simulink model "adaptivePIDv2"  (R2024a)
settings: Solver=ode45  StartTime=0.0  StopTime=5  FixedStep=1E-4  MaxStep=1E-4  RelTol=1E-3
values from neighbouring files (symbols this model uses):
  x = [input(1);input(2);input(3)]    [Dist_observer.m]
  y = [input(4),input(5),input(6)]'    [controller.m]
undefined symbols (not defined in the file or in its folder): initial_1, observer, z
settings Model: Creator=b_ant  LastModifiedBy=b_ant
settings SolverCC: ZeroCrossAlgorithm=Adaptive
settings DebuggingCC: IgnoredZcDiagnostic=none  UnconnectedInputMsg=warning  UnconnectedOutputMsg=warning  UnconnectedLineMsg=warning
settings ModelReferenceCC: EnableRefExpFcnMdlSchedulingChecks=on
settings RTWCC: GPUComputeCapability=3.5  DLArmComputeVersion=19.05

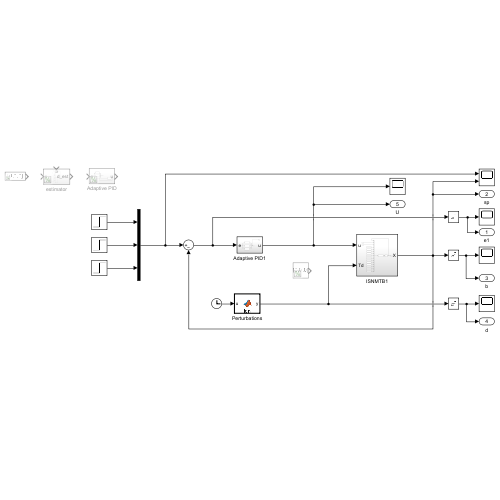
[thumbnail: Simulink's stored preview of the top-level diagram]
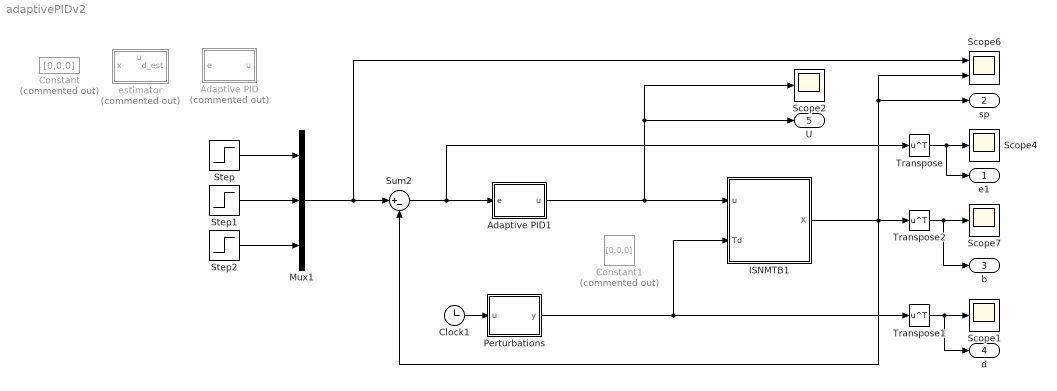
== system adaptivePIDv2 ==
  Adaptive PID : Subsystem  Commented=on
  Adaptive PID1 : Subsystem
  Clock1 : Clock
      settings: Decimation=1000
  Constant : Constant  Commented=on  Value=[0,0,0]
  Constant1 : Constant  Commented=on  Value=[0,0,0]
  ISNMTB1 : Subsystem
  Mux1 : Mux  Inputs=3
  Perturbations : MATLAB Function  TreatAsAtomicUnit=on
  Scope{1..2,4,7} (4 alike) : Scope
  Scope6 : Scope  NumInputPorts=2
  Step : Step  Time=0.1  SampleTime=0
  Step1 : Step  Time=0.1  SampleTime=0
  Step2 : Step  Time=0.1  SampleTime=0
  Sum2 : Sum  Inputs=|+-
  Transpose : Math  Operator=transpose
  Transpose1 : Math  Operator=transpose
  Transpose2 : Math  Operator=transpose
  estimator : Subsystem  Commented=on
      settings: PortSchema="{\"entries\":[{\"content\":{\"sides\":[{\"content\":{\"connectorIds\":[\"In1\"]},\"type\":\"ConnectorPlacement.EquallySpacedRectSide\",\"uuid\":\"f9e844d6-ee13-4ae8-8d73-084dc6b9c230\"},{\"content\":{\"connectorIds\":[\"Out1\"],\"side\":\"RIGHT\"},\"type\":\"ConnectorPlacement.EquallySpacedRectSide\",\"uuid\":\"c081e574-2129-4344-8b67-56cd55c23b50\"},{\"content\":{\"connectorIds\":[\"In2\"],\"side\":\"TOP\"},\"type\":\"ConnectorPlacement.EquallySpacedRectSide\",\"uuid\":\"bf6f2985-e51e-41d0-a8b1-b5505659e5f3\"},{\"content\":{\"side\":\"BOTTOM\"},\"type\":\"ConnectorPlacement.EquallySpacedRectSide\",\"uuid\":\"e1697b77-960b-449d-843b-5909cf972339\"}]},\"type\":\"ConnectorPlacement.EquallySpacedConnector\",\"uuid\":\"c9da1c41-5311-41bf-ab5b-06506202d90f\"}],\"packageUris\":[\"http://schema.mathworks.com/mf0/Connector/R2020b\"],\"version\":\"1.0\"}"
  e1 : Outport
  sp : Outport  Port=2
  b : Outport  Port=3
  d : Outport  Port=4
  U : Outport  Port=5
  wires:
  Transpose1/1 -> Scope1/1, d/1
  ISNMTB1/1(X) -> sp/1, Scope6/2, Sum2/2, Transpose2/1
  Sum2/1 -> Transpose/1, Adaptive PID1/1(e)
  Step2/1 -> Mux1/3
  Transpose2/1 -> Scope7/1, b/1
  Step1/1 -> Mux1/2
  Clock1/1 -> Perturbations/1(u)
  Transpose/1 -> e1/1, Scope4/1
  Step/1 -> Mux1/1
  Mux1/1 -> Sum2/1, Scope6/1
  Perturbations/1(y) -> ISNMTB1/2(Td), Transpose1/1
  Adaptive PID1/1(u) -> U/1, Scope2/1, ISNMTB1/1(u)

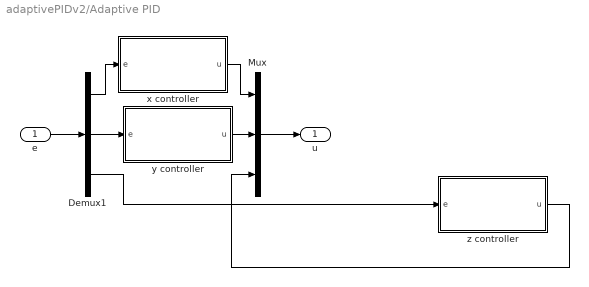
== system adaptivePIDv2/Adaptive PID ==
  e : Inport
  Demux1 : Demux  Outputs=3
  Mux : Mux  Inputs=3
  x controller : Subsystem
  y controller : Subsystem
  z controller : Subsystem
  u : Outport
  wires:
  z controller/1(u) -> Mux/3
  Demux1/2 -> y controller/1(e)
  x controller/1(u) -> Mux/1
  e/1 -> Demux1/1
  y controller/1(u) -> Mux/2
  Demux1/3 -> z controller/1(e)
  Demux1/1 -> x controller/1(e)
  Mux/1 -> u/1

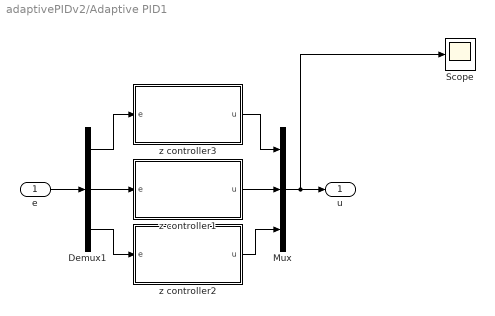
== system adaptivePIDv2/Adaptive PID1 ==
  e : Inport
  Demux1 : Demux  Outputs=3
  Mux : Mux  Inputs=3
  Scope : Scope
  z controller1 : Subsystem
  z controller2 : Subsystem
  z controller3 : Subsystem
  u : Outport
  wires:
  Demux1/2 -> z controller1/1(e)
  z controller3/1(u) -> Mux/1
  e/1 -> Demux1/1
  Demux1/1 -> z controller3/1(e)
  Mux/1 -> Scope/1, u/1
  Demux1/3 -> z controller2/1(e)
  z controller1/1(u) -> Mux/2
  z controller2/1(u) -> Mux/3

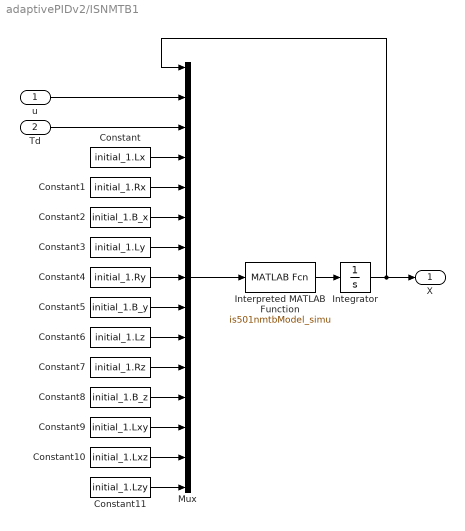
== system adaptivePIDv2/ISNMTB1 ==
  u : Inport
  Td : Inport  Port=2
  Constant : Constant  Value=initial_1.Lx
  Constant1 : Constant  Value=initial_1.Rx
  Constant10 : Constant  Value=initial_1.Lxz
  Constant11 : Constant  Value=initial_1.Lzy
  Constant2 : Constant  Value=initial_1.B_x
  Constant3 : Constant  Value=initial_1.Ly
  Constant4 : Constant  Value=initial_1.Ry
  Constant5 : Constant  Value=initial_1.B_y
  Constant6 : Constant  Value=initial_1.Lz
  Constant7 : Constant  Value=initial_1.Rz
  Constant8 : Constant  Value=initial_1.B_z
  Constant9 : Constant  Value=initial_1.Lxy
  Integrator : Integrator  InitialCondition=[3.249E4, -2.265E4, 3.655E4]
  Interpreted MATLAB Function : MATLABFcn  MATLABFcn=is501nmtbModel_simu
  Mux : Mux  Inputs=15
  X : Outport
  wires:
  Interpreted MATLAB Function/1 -> Integrator/1
  Integrator/1 -> X/1, Mux/1
  Mux/1 -> Interpreted MATLAB Function/1
  u/1 -> Mux/2
  Td/1 -> Mux/3
  Constant/1 -> Mux/4
  Constant1/1 -> Mux/5
  Constant2/1 -> Mux/6
  Constant3/1 -> Mux/7
  Constant4/1 -> Mux/8
  Constant5/1 -> Mux/9
  Constant6/1 -> Mux/10
  Constant7/1 -> Mux/11
  Constant8/1 -> Mux/12
  Constant9/1 -> Mux/13
  Constant10/1 -> Mux/14
  Constant11/1 -> Mux/15

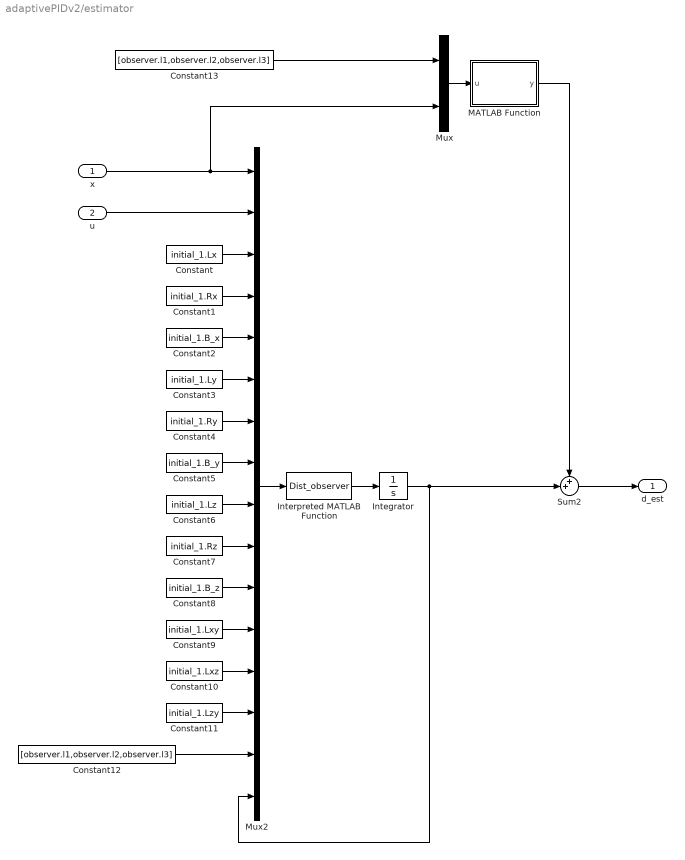
== system adaptivePIDv2/estimator ==
  x : Inport
  u : Inport  Port=2
  Constant : Constant  Value=initial_1.Lx
  Constant1 : Constant  Value=initial_1.Rx
  Constant10 : Constant  Value=initial_1.Lxz
  Constant11 : Constant  Value=initial_1.Lzy
  Constant12 : Constant  Value=[observer.l1,observer.l2,observer.l3]
  Constant13 : Constant  Value=[observer.l1,observer.l2,observer.l3]
  Constant2 : Constant  Value=initial_1.B_x
  Constant3 : Constant  Value=initial_1.Ly
  Constant4 : Constant  Value=initial_1.Ry
  Constant5 : Constant  Value=initial_1.B_y
  Constant6 : Constant  Value=initial_1.Lz
  Constant7 : Constant  Value=initial_1.Rz
  Constant8 : Constant  Value=initial_1.B_z
  Constant9 : Constant  Value=initial_1.Lxy
  Integrator : Integrator  InitialCondition=[0,0,0]
  Interpreted MATLAB Function : MATLABFcn  MATLABFcn=Dist_observer
  MATLAB Function : MATLAB Function  TreatAsAtomicUnit=on
  Mux : Mux  Inputs=2
  Mux2 : Mux  Inputs=16
  Sum2 : Sum  Inputs=++|
  d_est : Outport
  wires:
  Constant6/1 -> Mux2/9
  MATLAB Function/1(y) -> Sum2/1
  Constant10/1 -> Mux2/13
  Integrator/1 -> Sum2/2, Mux2/16
  Interpreted MATLAB Function/1 -> Integrator/1
  Constant2/1 -> Mux2/5
  Constant4/1 -> Mux2/7
  Constant7/1 -> Mux2/10
  Mux2/1 -> Interpreted MATLAB Function/1
  Constant11/1 -> Mux2/14
  Constant8/1 -> Mux2/11
  Constant1/1 -> Mux2/4
  Constant3/1 -> Mux2/6
  Constant/1 -> Mux2/3
  Constant9/1 -> Mux2/12
  Constant5/1 -> Mux2/8
  Constant12/1 -> Mux2/15
  u/1 -> Mux2/2
  Sum2/1 -> d_est/1
  Constant13/1 -> Mux/1
  Mux/1 -> MATLAB Function/1(u)
  x/1 -> Mux/2, Mux2/1

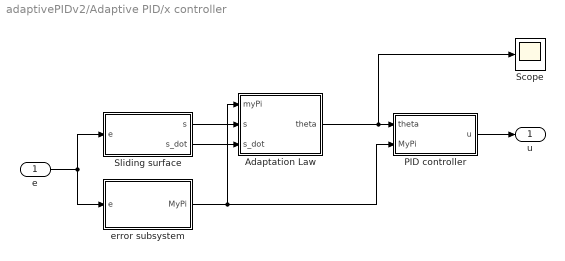
== system adaptivePIDv2/Adaptive PID/x controller ==
  e : Inport
  Adaptation Law : Subsystem  mask{alpha=x.alpha, beta=x.beta, epsilon=x.epsilon, n=x.n, kd0=x.kd_init, ki0=x.ki_init, kp0=x.kp_init}
      mask prompts: kd0 "kd_0:"; ki0 "ki_0:"; kp0 "kp_0:"
      mask TypeOptions alpha: alpha/Value
      mask TypeOptions beta: beta/Value
      mask TypeOptions epsilon: epsilon/Value
      mask TypeOptions n: n/Value
      mask TypeOptions kd0: kd0/Value
      mask TypeOptions ki0: ki0/Value
      mask TypeOptions kp0: kp0/Value
  PID controller : Subsystem
  Scope : Scope
  Sliding surface : Subsystem  mask{Gain=x.lambda}
      mask prompts: Gain "Simulink:blkprm_prompts:GainGain"
      mask TypeOptions Gain: Gain/Gain
      mask DialogControl Gain Prompt: Gain:
  error subsystem : Subsystem
  u : Outport
  wires:
  Sliding surface/1(s) -> Adaptation Law/2(s)
  Sliding surface/2(s_dot) -> Adaptation Law/3(s_dot)
  PID controller/1(u) -> u/1
  error subsystem/1(MyPi) -> PID controller/2(MyPi), Adaptation Law/1(myPi)
  e/1 -> Sliding surface/1(e), error subsystem/1(e)
  Adaptation Law/1(theta) -> Scope/1, PID controller/1(theta)

== system adaptivePIDv2/Adaptive PID/y controller ==
  e : Inport
  Adaptation Law : Subsystem  mask{alpha=y.alpha, beta=y.beta, epsilon=y.epsilon, n=y.n, kd0=y.kd_init, ki0=y.ki_init, kp0=y.kp_init}
      mask prompts: kd0 "kd_0:"; ki0 "ki_0:"; kp0 "kp_0:"
      mask TypeOptions alpha: alpha/Value
      mask TypeOptions beta: beta/Value
      mask TypeOptions epsilon: epsilon/Value
      mask TypeOptions n: n/Value
      mask TypeOptions kd0: kd0/Value
      mask TypeOptions ki0: ki0/Value
      mask TypeOptions kp0: kp0/Value
  PID controller : Subsystem
  Scope : Scope
  Sliding surface : Subsystem  mask{Gain=y.lambda}
      mask prompts: Gain "Simulink:blkprm_prompts:GainGain"
      mask TypeOptions Gain: Gain/Gain
      mask DialogControl Gain Prompt: Gain:
  error subsystem : Subsystem
  u : Outport
  wires:
  e/1 -> Sliding surface/1(e), error subsystem/1(e)
  error subsystem/1(MyPi) -> Adaptation Law/1(myPi), PID controller/2(MyPi)
  Adaptation Law/1(theta) -> PID controller/1(theta), Scope/1
  PID controller/1(u) -> u/1
  Sliding surface/2(s_dot) -> Adaptation Law/3(s_dot)
  Sliding surface/1(s) -> Adaptation Law/2(s)

== system adaptivePIDv2/Adaptive PID/z controller ==
  e : Inport
  Adaptation Law : Subsystem  mask{alpha=z.alpha, beta=z.beta, epsilon=z.epsilon, n=z.n, kd0=z.kd_init, ki0=z.ki_init, kp0=z.kp_init}
      mask prompts: kd0 "kd_0:"; ki0 "ki_0:"; kp0 "kp_0:"
      mask TypeOptions alpha: alpha/Value
      mask TypeOptions beta: beta/Value
      mask TypeOptions epsilon: epsilon/Value
      mask TypeOptions n: n/Value
      mask TypeOptions kd0: kd0/Value
      mask TypeOptions ki0: ki0/Value
      mask TypeOptions kp0: kp0/Value
  PID controller : Subsystem
  Scope : Scope
  Sliding surface : Subsystem  mask{Gain=z.lambda}
      mask prompts: Gain "Simulink:blkprm_prompts:GainGain"
      mask TypeOptions Gain: Gain/Gain
      mask DialogControl Gain Prompt: Gain:
  error subsystem : Subsystem
  u : Outport
  wires:
  Sliding surface/1(s) -> Adaptation Law/2(s)
  Sliding surface/2(s_dot) -> Adaptation Law/3(s_dot)
  PID controller/1(u) -> u/1
  Adaptation Law/1(theta) -> Scope/1, PID controller/1(theta)
  error subsystem/1(MyPi) -> PID controller/2(MyPi), Adaptation Law/1(myPi)
  e/1 -> error subsystem/1(e), Sliding surface/1(e)

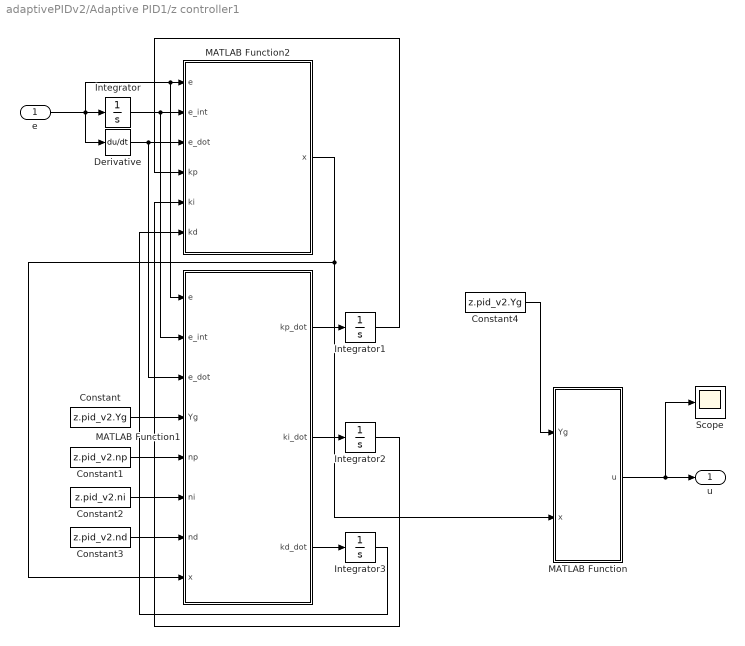
== system adaptivePIDv2/Adaptive PID1/z controller1 ==
  e : Inport
  Constant : Constant  Value=z.pid_v2.Yg
  Constant1 : Constant  Value=z.pid_v2.np
  Constant2 : Constant  Value=z.pid_v2.ni
  Constant3 : Constant  Value=z.pid_v2.nd
  Constant4 : Constant  Value=z.pid_v2.Yg
  Derivative : Derivative
  Integrator : Integrator
  Integrator1 : Integrator  InitialCondition=y.PID.Kp
  Integrator2 : Integrator  InitialCondition=y.PID.Ki
  Integrator3 : Integrator  InitialCondition=y.PID.Kd
  MATLAB Function : MATLAB Function  TreatAsAtomicUnit=on
  MATLAB Function1 : MATLAB Function  TreatAsAtomicUnit=on
  MATLAB Function2 : MATLAB Function  TreatAsAtomicUnit=on
  Scope : Scope
  u : Outport
  wires:
  e/1 -> Derivative/1, Integrator/1, MATLAB Function1/1(e), MATLAB Function2/1(e)
  Constant/1 -> MATLAB Function1/4(Yg)
  Constant1/1 -> MATLAB Function1/5(np)
  Constant2/1 -> MATLAB Function1/6(ni)
  Constant3/1 -> MATLAB Function1/7(nd)
  Constant4/1 -> MATLAB Function/1(Yg)
  MATLAB Function1/1(kp_dot) -> Integrator1/1
  MATLAB Function1/2(ki_dot) -> Integrator2/1
  MATLAB Function1/3(kd_dot) -> Integrator3/1
  Integrator/1 -> MATLAB Function1/2(e_int), MATLAB Function2/2(e_int)
  Derivative/1 -> MATLAB Function1/3(e_dot), MATLAB Function2/3(e_dot)
  MATLAB Function2/1(x) -> MATLAB Function/2(x), MATLAB Function1/8(x)
  Integrator1/1 -> MATLAB Function2/4(kp)
  Integrator2/1 -> MATLAB Function2/5(ki)
  Integrator3/1 -> MATLAB Function2/6(kd)
  MATLAB Function/1(u) -> Scope/1, u/1

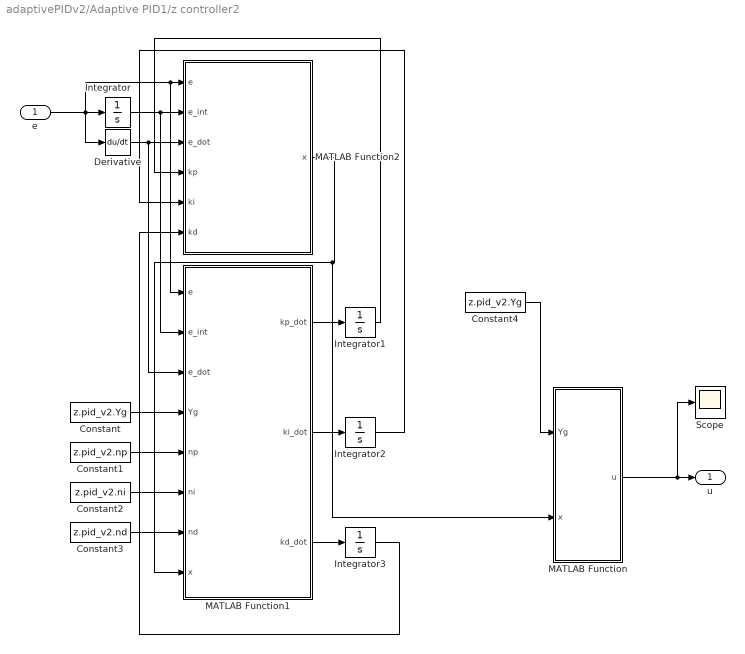
== system adaptivePIDv2/Adaptive PID1/z controller2 ==
  e : Inport
  Constant : Constant  Value=z.pid_v2.Yg
  Constant1 : Constant  Value=z.pid_v2.np
  Constant2 : Constant  Value=z.pid_v2.ni
  Constant3 : Constant  Value=z.pid_v2.nd
  Constant4 : Constant  Value=z.pid_v2.Yg
  Derivative : Derivative
  Integrator : Integrator
  Integrator1 : Integrator  InitialCondition=z.PID.Kp
  Integrator2 : Integrator  InitialCondition=z.PID.Ki
  Integrator3 : Integrator  InitialCondition=z.PID.Kd
  MATLAB Function : MATLAB Function  TreatAsAtomicUnit=on
  MATLAB Function1 : MATLAB Function  TreatAsAtomicUnit=on
  MATLAB Function2 : MATLAB Function  TreatAsAtomicUnit=on
  Scope : Scope
  u : Outport
  wires:
  e/1 -> Derivative/1, Integrator/1, MATLAB Function1/1(e), MATLAB Function2/1(e)
  Constant/1 -> MATLAB Function1/4(Yg)
  Constant1/1 -> MATLAB Function1/5(np)
  Constant2/1 -> MATLAB Function1/6(ni)
  Constant3/1 -> MATLAB Function1/7(nd)
  Constant4/1 -> MATLAB Function/1(Yg)
  MATLAB Function1/1(kp_dot) -> Integrator1/1
  MATLAB Function1/2(ki_dot) -> Integrator2/1
  MATLAB Function1/3(kd_dot) -> Integrator3/1
  Integrator/1 -> MATLAB Function1/2(e_int), MATLAB Function2/2(e_int)
  Derivative/1 -> MATLAB Function1/3(e_dot), MATLAB Function2/3(e_dot)
  MATLAB Function2/1(x) -> MATLAB Function/2(x), MATLAB Function1/8(x)
  Integrator1/1 -> MATLAB Function2/4(kp)
  Integrator2/1 -> MATLAB Function2/5(ki)
  Integrator3/1 -> MATLAB Function2/6(kd)
  MATLAB Function/1(u) -> Scope/1, u/1

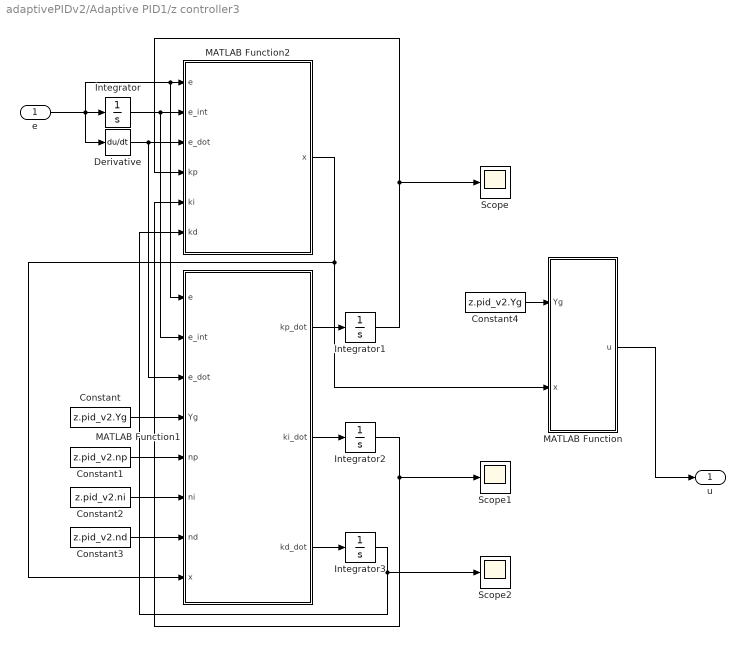
== system adaptivePIDv2/Adaptive PID1/z controller3 ==
  e : Inport
  Constant : Constant  Value=z.pid_v2.Yg
  Constant1 : Constant  Value=z.pid_v2.np
  Constant2 : Constant  Value=z.pid_v2.ni
  Constant3 : Constant  Value=z.pid_v2.nd
  Constant4 : Constant  Value=z.pid_v2.Yg
  Derivative : Derivative
  Integrator : Integrator
  Integrator1 : Integrator  InitialCondition=x.PID.Kp
  Integrator2 : Integrator  InitialCondition=x.PID.Ki
  Integrator3 : Integrator  InitialCondition=x.PID.Kd
  MATLAB Function : MATLAB Function  TreatAsAtomicUnit=on
  MATLAB Function1 : MATLAB Function  TreatAsAtomicUnit=on
  MATLAB Function2 : MATLAB Function  TreatAsAtomicUnit=on
  Scope : Scope
  Scope1 : Scope
  Scope2 : Scope
  u : Outport
  wires:
  e/1 -> Derivative/1, Integrator/1, MATLAB Function1/1(e), MATLAB Function2/1(e)
  Constant/1 -> MATLAB Function1/4(Yg)
  Constant1/1 -> MATLAB Function1/5(np)
  Constant2/1 -> MATLAB Function1/6(ni)
  Constant3/1 -> MATLAB Function1/7(nd)
  Constant4/1 -> MATLAB Function/1(Yg)
  MATLAB Function1/1(kp_dot) -> Integrator1/1
  MATLAB Function1/2(ki_dot) -> Integrator2/1
  MATLAB Function1/3(kd_dot) -> Integrator3/1
  Integrator/1 -> MATLAB Function1/2(e_int), MATLAB Function2/2(e_int)
  Derivative/1 -> MATLAB Function1/3(e_dot), MATLAB Function2/3(e_dot)
  MATLAB Function2/1(x) -> MATLAB Function/2(x), MATLAB Function1/8(x)
  Integrator1/1 -> Scope/1, MATLAB Function2/4(kp)
  Integrator2/1 -> MATLAB Function2/5(ki), Scope1/1
  Integrator3/1 -> Scope2/1, MATLAB Function2/6(kd)
  MATLAB Function/1(u) -> u/1

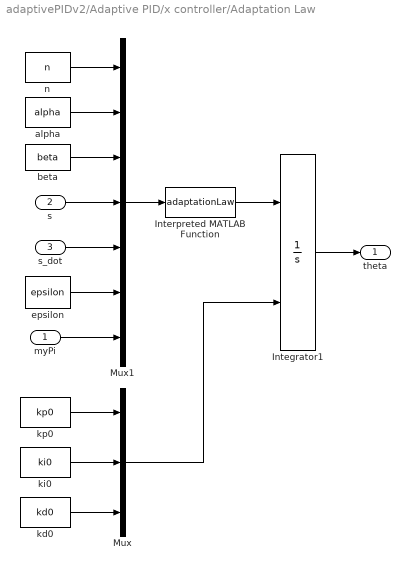
== system adaptivePIDv2/Adaptive PID/x controller/Adaptation Law ==
  myPi : Inport
  s : Inport  Port=2
  s_dot : Inport  Port=3
  Integrator1 : Integrator  InitialConditionSource=external  InitialCondition=[1.460477259865257e-04,6.548069875818259e-05,0]
  Interpreted MATLAB Function : MATLABFcn  MATLABFcn=adaptationLaw
  Mux : Mux  Inputs=3
  Mux1 : Mux  Inputs=7
  alpha : Constant  Value=alpha
  beta : Constant  Value=beta
  epsilon : Constant  Value=epsilon
  kd0 : Constant  Value=kd0
  ki0 : Constant  Value=ki0
  kp0 : Constant  Value=kp0
  n : Constant  Value=n
  theta : Outport
  wires:
  alpha/1 -> Mux1/2
  Interpreted MATLAB Function/1 -> Integrator1/1
  myPi/1 -> Mux1/7
  s/1 -> Mux1/4
  epsilon/1 -> Mux1/6
  Integrator1/1 -> theta/1
  s_dot/1 -> Mux1/5
  beta/1 -> Mux1/3
  Mux1/1 -> Interpreted MATLAB Function/1
  n/1 -> Mux1/1
  ki0/1 -> Mux/2
  Mux/1 -> Integrator1/2
  kp0/1 -> Mux/1
  kd0/1 -> Mux/3

== system adaptivePIDv2/Adaptive PID/x controller/PID controller ==
  theta : Inport
  MyPi : Inport  Port=2
  Interpreted MATLAB Function1 : MATLABFcn  MATLABFcn=controlLaw  OutputDimensions=1
  Mux2 : Mux  Inputs=2
  u : Outport
  wires:
  Mux2/1 -> Interpreted MATLAB Function1/1
  theta/1 -> Mux2/1
  Interpreted MATLAB Function1/1 -> u/1
  MyPi/1 -> Mux2/2

== system adaptivePIDv2/Adaptive PID/x controller/Sliding surface ==
  note: s
  note: e
  e : Inport
  Add : Sum
  Derivative : Derivative
  Derivative1 : Derivative
  Gain : Gain  Gain=Gain
  s : Outport
  s_dot : Outport  Port=2
  wires:
  Add/1 -> s/1, Derivative/1
  Gain/1 -> Add/1
  e/1 -> Derivative1/1, Gain/1
  Derivative1/1 -> Add/2
  Derivative/1 -> s_dot/1

== system adaptivePIDv2/Adaptive PID/x controller/error subsystem ==
  e : Inport
  Derivative : Derivative
  Integrator : Integrator
  Mux : Mux  Inputs=3
  MyPi : Outport
  wires:
  e/1 -> Derivative/1, Mux/1, Integrator/1
  Integrator/1 -> Mux/2
  Mux/1 -> MyPi/1
  Derivative/1 -> Mux/3

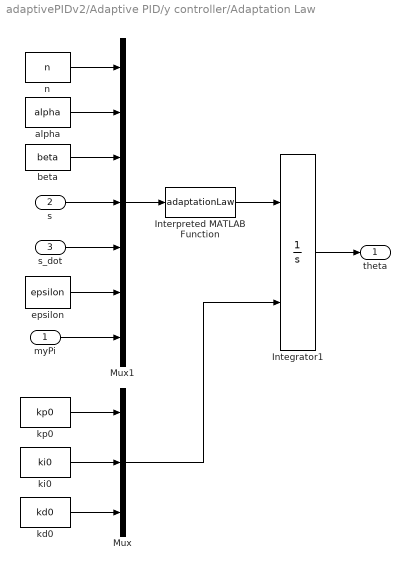
== system adaptivePIDv2/Adaptive PID/y controller/Adaptation Law ==
  myPi : Inport
  s : Inport  Port=2
  s_dot : Inport  Port=3
  Integrator1 : Integrator  InitialConditionSource=external  InitialCondition=[1.460477259865257e-04,6.548069875818259e-05,0]
  Interpreted MATLAB Function : MATLABFcn  MATLABFcn=adaptationLaw
  Mux : Mux  Inputs=3
  Mux1 : Mux  Inputs=7
  alpha : Constant  Value=alpha
  beta : Constant  Value=beta
  epsilon : Constant  Value=epsilon
  kd0 : Constant  Value=kd0
  ki0 : Constant  Value=ki0
  kp0 : Constant  Value=kp0
  n : Constant  Value=n
  theta : Outport
  wires:
  kd0/1 -> Mux/3
  kp0/1 -> Mux/1
  Mux/1 -> Integrator1/2
  ki0/1 -> Mux/2
  n/1 -> Mux1/1
  Mux1/1 -> Interpreted MATLAB Function/1
  beta/1 -> Mux1/3
  s_dot/1 -> Mux1/5
  Integrator1/1 -> theta/1
  epsilon/1 -> Mux1/6
  s/1 -> Mux1/4
  myPi/1 -> Mux1/7
  Interpreted MATLAB Function/1 -> Integrator1/1
  alpha/1 -> Mux1/2

== system adaptivePIDv2/Adaptive PID/y controller/PID controller ==
  theta : Inport
  MyPi : Inport  Port=2
  Interpreted MATLAB Function1 : MATLABFcn  MATLABFcn=controlLaw  OutputDimensions=1
  Mux2 : Mux  Inputs=2
  u : Outport
  wires:
  MyPi/1 -> Mux2/2
  Interpreted MATLAB Function1/1 -> u/1
  theta/1 -> Mux2/1
  Mux2/1 -> Interpreted MATLAB Function1/1

== system adaptivePIDv2/Adaptive PID/y controller/Sliding surface ==
  note: e
  note: s
  e : Inport
  Add : Sum
  Derivative : Derivative
  Derivative1 : Derivative
  Gain : Gain  Gain=Gain
  s : Outport
  s_dot : Outport  Port=2
  wires:
  Derivative/1 -> s_dot/1
  Derivative1/1 -> Add/2
  e/1 -> Derivative1/1, Gain/1
  Gain/1 -> Add/1
  Add/1 -> s/1, Derivative/1

== system adaptivePIDv2/Adaptive PID/y controller/error subsystem ==
  e : Inport
  Derivative : Derivative
  Integrator : Integrator
  Mux : Mux  Inputs=3
  MyPi : Outport
  wires:
  Derivative/1 -> Mux/3
  Mux/1 -> MyPi/1
  Integrator/1 -> Mux/2
  e/1 -> Derivative/1, Integrator/1, Mux/1

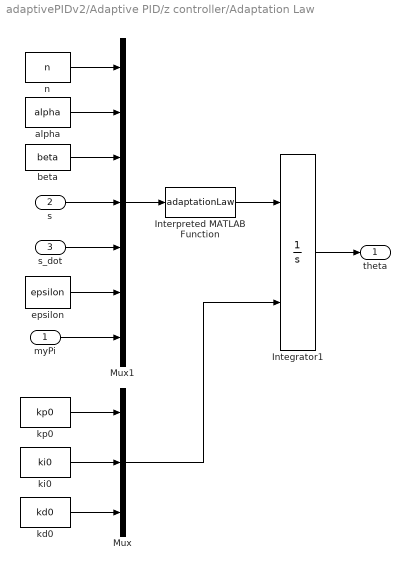
== system adaptivePIDv2/Adaptive PID/z controller/Adaptation Law ==
  myPi : Inport
  s : Inport  Port=2
  s_dot : Inport  Port=3
  Integrator1 : Integrator  InitialConditionSource=external  InitialCondition=[1.460477259865257e-04,6.548069875818259e-05,0]
  Interpreted MATLAB Function : MATLABFcn  MATLABFcn=adaptationLaw
  Mux : Mux  Inputs=3
  Mux1 : Mux  Inputs=7
  alpha : Constant  Value=alpha
  beta : Constant  Value=beta
  epsilon : Constant  Value=epsilon
  kd0 : Constant  Value=kd0
  ki0 : Constant  Value=ki0
  kp0 : Constant  Value=kp0
  n : Constant  Value=n
  theta : Outport
  wires:
  alpha/1 -> Mux1/2
  Interpreted MATLAB Function/1 -> Integrator1/1
  myPi/1 -> Mux1/7
  s/1 -> Mux1/4
  epsilon/1 -> Mux1/6
  Integrator1/1 -> theta/1
  s_dot/1 -> Mux1/5
  beta/1 -> Mux1/3
  Mux1/1 -> Interpreted MATLAB Function/1
  n/1 -> Mux1/1
  ki0/1 -> Mux/2
  Mux/1 -> Integrator1/2
  kp0/1 -> Mux/1
  kd0/1 -> Mux/3

== system adaptivePIDv2/Adaptive PID/z controller/PID controller ==
  theta : Inport
  MyPi : Inport  Port=2
  Interpreted MATLAB Function1 : MATLABFcn  MATLABFcn=controlLaw  OutputDimensions=1
  Mux2 : Mux  Inputs=2
  u : Outport
  wires:
  Mux2/1 -> Interpreted MATLAB Function1/1
  theta/1 -> Mux2/1
  Interpreted MATLAB Function1/1 -> u/1
  MyPi/1 -> Mux2/2

== system adaptivePIDv2/Adaptive PID/z controller/Sliding surface ==
  note: s
  note: e
  e : Inport
  Add : Sum
  Derivative : Derivative
  Derivative1 : Derivative
  Gain : Gain  Gain=Gain
  s : Outport
  s_dot : Outport  Port=2
  wires:
  Add/1 -> s/1, Derivative/1
  Gain/1 -> Add/1
  e/1 -> Derivative1/1, Gain/1
  Derivative1/1 -> Add/2
  Derivative/1 -> s_dot/1

== system adaptivePIDv2/Adaptive PID/z controller/error subsystem ==
  e : Inport
  Derivative : Derivative
  Integrator : Integrator
  Mux : Mux  Inputs=3
  MyPi : Outport
  wires:
  e/1 -> Derivative/1, Mux/1, Integrator/1
  Integrator/1 -> Mux/2
  Mux/1 -> MyPi/1
  Derivative/1 -> Mux/3

== matlab function adaptivePIDv2/Adaptive PID1/z controller3/MATLAB Function2 ==
  data: e input; x output; e_int input; e_dot input; kp input; ki input; kd input
function x = myPidFun(e,e_int,e_dot,kp,ki,kd)
   x = kp*e+ki*e_int+kd*e_dot;
end

== matlab function adaptivePIDv2/Adaptive PID1/z controller2/MATLAB Function1 ==
  data: e input; kp_dot output; e_int input; e_dot input; Yg input; np input; ni input; nd input; ki_dot output; kd_dot output; x input
function [kp_dot,ki_dot,kd_dot] = neuronalPID(e,e_int,e_dot,Yg,np,ni,nd,x)
%e = entr(1);
%e_int = entr(2);
%e_dot = entr(3);
%x =  entr(4);
%Yg =  entr(5);
%np =  entr(6);
%ni =  entr(7);
%nd =  entr(8);
%kp_old
%ki_old
%kd_old 

kp_dot = np*e*e*sigmoid_dot(x, Yg);
ki_dot = ni*e*e_int*sigmoid_dot(x, Yg);
kd_dot = nd*e*e_dot*sigmoid_dot(x, Yg);
end

function f_dot = sigmoid_dot(x, Yg)
    f_dot = 4*exp(-x*Yg)/(1+exp(-x*Yg))^2;
end

== matlab function adaptivePIDv2/Adaptive PID1/z controller2/MATLAB Function2 ==
  data: e input; x output; e_int input; e_dot input; kp input; ki input; kd input
function x = myPidFun(e,e_int,e_dot,kp,ki,kd)
   x = kp*e+ki*e_int+kd*e_dot;
end

== matlab function adaptivePIDv2/Perturbations ==
  data: u input; y output
function y = fcn(u)
y= [2.522*sin(2*pi*4.788E-3*u)+3.249E04;
   -5.174*sin(2*pi*7.481E-3*u)-2.265E04;
    3.359*sin(2*pi*8.378E-3*u)+3.655E04];
end

== matlab function adaptivePIDv2/Adaptive PID1/z controller1/MATLAB Function ==
  data: Yg input; u output; x input
function u = fcn(Yg, x)
    u=sigmoid(x,Yg);
end

function f = sigmoid(x,Yg)
    f = 2/Yg * (1-exp(-x*Yg))/(1+exp(-x*Yg));
end

== matlab function adaptivePIDv2/estimator/MATLAB Function ==
  data: u input; y output
function y = fcn(u)
l = diag([u(1),u(2),u(3)]);
x = [u(4);u(5);u(6)];

y = l*x;
end

== matlab function adaptivePIDv2/Adaptive PID1/z controller1/MATLAB Function1 ==
  data: e input; kp_dot output; e_int input; e_dot input; Yg input; np input; ni input; nd input; ki_dot output; kd_dot output; x input
function [kp_dot,ki_dot,kd_dot] = neuronalPID(e,e_int,e_dot,Yg,np,ni,nd,x)
%e = entr(1);
%e_int = entr(2);
%e_dot = entr(3);
%x =  entr(4);
%Yg =  entr(5);
%np =  entr(6);
%ni =  entr(7);
%nd =  entr(8);
%kp_old
%ki_old
%kd_old 

kp_dot = np*e*e*sigmoid_dot(x, Yg);
ki_dot = ni*e*e_int*sigmoid_dot(x, Yg);
kd_dot = nd*e*e_dot*sigmoid_dot(x, Yg);
end

function f_dot = sigmoid_dot(x, Yg)
    f_dot = 4*exp(-x*Yg)/(1+exp(-x*Yg))^2;
end

== matlab function adaptivePIDv2/Adaptive PID1/z controller3/MATLAB Function ==
  data: Yg input; u output; x input
function u = fcn(Yg, x)
    u=sigmoid(x,Yg);
end

function f = sigmoid(x,Yg)
    f = 2/Yg * (1-exp(-x*Yg))/(1+exp(-x*Yg));
end

== matlab function adaptivePIDv2/Adaptive PID1/z controller3/MATLAB Function1 ==
  data: e input; kp_dot output; e_int input; e_dot input; Yg input; np input; ni input; nd input; ki_dot output; kd_dot output; x input
function [kp_dot,ki_dot,kd_dot] = neuronalPID(e,e_int,e_dot,Yg,np,ni,nd,x)
%e = entr(1);
%e_int = entr(2);
%e_dot = entr(3);
%x =  entr(4);
%Yg =  entr(5);
%np =  entr(6);
%ni =  entr(7);
%nd =  entr(8);
%kp_old
%ki_old
%kd_old 

kp_dot = np*e*e*sigmoid_dot(x, Yg);
ki_dot = ni*e*e_int*sigmoid_dot(x, Yg);
kd_dot = nd*e*e_dot*sigmoid_dot(x, Yg);
end

function f_dot = sigmoid_dot(x, Yg)
    f_dot = 4*exp(-x*Yg)/(1+exp(-x*Yg))^2;
end

== matlab function adaptivePIDv2/Adaptive PID1/z controller1/MATLAB Function2 ==
  data: e input; x output; e_int input; e_dot input; kp input; ki input; kd input
function x = myPidFun(e,e_int,e_dot,kp,ki,kd)
   x = kp*e+ki*e_int+kd*e_dot;
end

== matlab function adaptivePIDv2/Adaptive PID1/z controller2/MATLAB Function ==
  data: Yg input; u output; x input
function u = fcn(Yg, x)
    u=sigmoid(x,Yg);
end

function f = sigmoid(x,Yg)
    f = 2/Yg * (1-exp(-x*Yg))/(1+exp(-x*Yg));
end
